simulink subsystem "Publish_Control_System_Out"  (R2023a)
settings: Solver=VariableStepAuto  StartTime=0.0  StopTime=10.0  RelTol=1e-3
undefined symbols (not defined in the file or in its folder): angular, data, data_SL_Info, linear
libraries: ros2lib x14
settings Model: Creator=hollis  LastModifiedBy=john

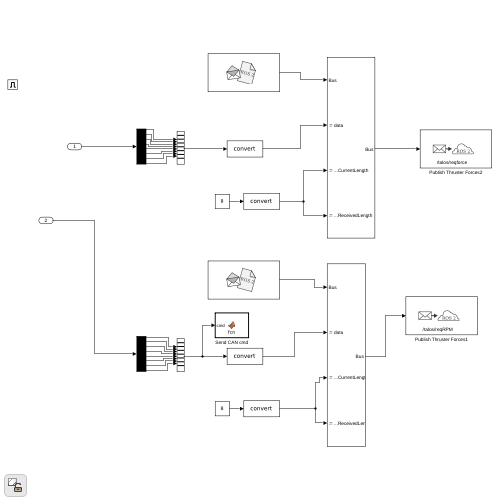
[thumbnail: Simulink's stored preview of the top-level diagram]
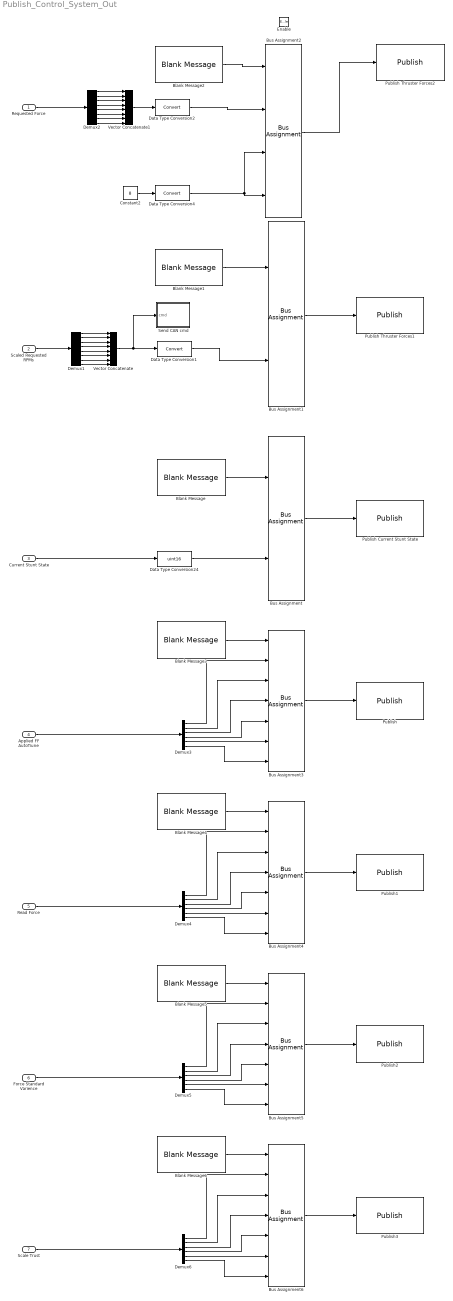
== system Publish_Control_System_Out ==
  Requested Force : Inport
  Scaled Requested RPMs : Inport  Port=2
  Current Stunt State : Inport  Port=3
  Applied FF AutoTiune : Inport  Port=4
  Read Force : Inport  Port=5
  Force Standard Varience : Inport  Port=6
  Scale Trust : Inport  Port=7
  Enable : EnablePort
  Blank Message : ros2lib/Blank Message  messageClass=Message  entityType=std_msgs/UInt16  messageType=std_msgs/UInt16  SampleTime=inf
  Blank Message1 : ros2lib/Blank Message  messageClass=Message  entityType=riptide_msgs2/DshotCommand  messageType=riptide_msgs2/DshotCommand  SampleTime=inf
      settings: LibrarySourceBlock=roslib/ROS 2/Blank Message
  Blank Message2 : ros2lib/Blank Message  messageClass=Message  entityType=std_msgs/Float32MultiArray  messageType=std_msgs/Float32MultiArray  SampleTime=inf
      settings: LibrarySourceBlock=roslib/ROS 2/Blank Message
  Blank Message{3..6} (4 alike) : ros2lib/Blank Message  messageClass=Message  entityType=geometry_msgs/Twist  messageType=geometry_msgs/Twist  SampleTime=inf
  Bus Assignment : BusAssignment  AssignedSignals=data
  Bus Assignment1 : BusAssignment  AssignedSignals=values
  Bus Assignment2 : BusAssignment  AssignedSignals=data,data_SL_Info.CurrentLength,data_SL_Info.ReceivedLength
  Bus Assignment{3..6} (4 alike) : BusAssignment  AssignedSignals=linear.x,linear.y,linear.z,angular.x,angular.y,angular.z
  Constant2 : Constant  Value=8
  Data Type Conversion1 : DataTypeConversion  SaturateOnIntegerOverflow=off  RndMeth=Floor
  Data Type Conversion2 : DataTypeConversion  SaturateOnIntegerOverflow=off  RndMeth=Floor
  Data Type Conversion24 : DataTypeConversion  OutDataTypeStr=uint16  SaturateOnIntegerOverflow=off  RndMeth=Floor
  Data Type Conversion4 : DataTypeConversion  SaturateOnIntegerOverflow=off  RndMeth=Floor
  Demux1 : Demux  Outputs=8
  Demux2 : Demux  Outputs=8
  Demux{3..6} (4 alike) : Demux  Outputs=6
  Publish : ros2lib/Publish  topicSource=Specify your own  topic=/talos/ff_auto_tune  messageType=geometry_msgs/Twist  QOSHistory=Keep last  QOSDepth=1  QOSReliability=Reliable  QOSDurability=Volatile
  Publish Current Stunt State : ros2lib/Publish  topicSource=Specify your own  topic=/talos/controller/running_stunt_state  messageType=std_msgs/UInt16  QOSHistory=Keep last  QOSDepth=1  QOSReliability=Reliable  QOSDurability=Volatile
  Publish Thruster Forces1 : ros2lib/Publish  topicSource=Specify your own  topic=/talos/command/requested_rpm  messageType=riptide_msgs2/DshotCommand  QOSHistory=Keep last  QOSDepth=1  QOSReliability=Reliable  QOSDurability=Volatile
      settings: LibrarySourceBlock=roslib/ROS 2/Publish
  Publish Thruster Forces2 : ros2lib/Publish  topicSource=Specify your own  topic=/talos/thruster_forces  messageType=std_msgs/Float32MultiArray  QOSHistory=Keep last  QOSDepth=1  QOSReliability=Reliable  QOSDurability=Volatile
      settings: LibrarySourceBlock=roslib/ROS 2/Publish
  Publish1 : ros2lib/Publish  topicSource=Specify your own  topic=/talos/controller/scale/applied_force_reading  messageType=geometry_msgs/Twist  QOSHistory=Keep last  QOSDepth=1  QOSReliability=Reliable  QOSDurability=Volatile
  Publish2 : ros2lib/Publish  topicSource=Specify your own  topic=/talos/controller/scale/standard_variance  messageType=geometry_msgs/Twist  QOSHistory=Keep last  QOSDepth=1  QOSReliability=Reliable  QOSDurability=Volatile
  Publish3 : ros2lib/Publish  topicSource=Specify your own  topic=/talos/controller/scale/trust  messageType=geometry_msgs/Twist  QOSHistory=Keep last  QOSDepth=1  QOSReliability=Reliable  QOSDurability=Volatile
  Send CAN cmd : MATLAB Function  TreatAsAtomicUnit=on
  Vector Concatenate : Concatenate  NumInputs=8
  Vector Concatenate1 : Concatenate  NumInputs=8
  wires:
  Demux1/8 -> Vector Concatenate/8
  Data Type Conversion2/1 -> Bus Assignment2/2
  Demux1/1 -> Vector Concatenate/1
  Demux2/4 -> Vector Concatenate1/4
  Demux2/5 -> Vector Concatenate1/5
  Demux2/2 -> Vector Concatenate1/2
  Blank Message2/1 -> Bus Assignment2/1
  Demux2/7 -> Vector Concatenate1/7
  Demux1/2 -> Vector Concatenate/2
  Constant2/1 -> Data Type Conversion4/1
  Blank Message1/1 -> Bus Assignment1/1
  Demux2/3 -> Vector Concatenate1/3
  Demux1/6 -> Vector Concatenate/6
  Scaled Requested RPMs/1 -> Demux1/1
  Data Type Conversion4/1 -> Bus Assignment2/4, Bus Assignment2/3
  Vector Concatenate1/1 -> Data Type Conversion2/1
  Demux1/4 -> Vector Concatenate/4
  Vector Concatenate/1 -> Send CAN cmd/1(cmd), Data Type Conversion1/1
  Demux1/5 -> Vector Concatenate/5
  Demux1/3 -> Vector Concatenate/3
  Demux2/8 -> Vector Concatenate1/8
  Demux2/6 -> Vector Concatenate1/6
  Demux1/7 -> Vector Concatenate/7
  Bus Assignment1/1 -> Publish Thruster Forces1/1
  Requested Force/1 -> Demux2/1
  Data Type Conversion1/1 -> Bus Assignment1/2
  Demux2/1 -> Vector Concatenate1/1
  Blank Message/1 -> Bus Assignment/1
  Bus Assignment/1 -> Publish Current Stunt State/1
  Current Stunt State/1 -> Data Type Conversion24/1
  Data Type Conversion24/1 -> Bus Assignment/2
  Applied FF AutoTiune/1 -> Demux3/1
  Demux3/6 -> Bus Assignment3/7
  Blank Message3/1 -> Bus Assignment3/1
  Bus Assignment3/1 -> Publish/1
  Demux3/1 -> Bus Assignment3/2
  Demux3/2 -> Bus Assignment3/3
  Demux3/4 -> Bus Assignment3/5
  Demux3/5 -> Bus Assignment3/6
  Demux3/3 -> Bus Assignment3/4
  Read Force/1 -> Demux4/1
  Blank Message4/1 -> Bus Assignment4/1
  Demux4/6 -> Bus Assignment4/7
  Demux4/2 -> Bus Assignment4/3
  Bus Assignment4/1 -> Publish1/1
  Demux4/1 -> Bus Assignment4/2
  Demux4/4 -> Bus Assignment4/5
  Demux4/5 -> Bus Assignment4/6
  Demux4/3 -> Bus Assignment4/4
  Force Standard Varience/1 -> Demux5/1
  Blank Message5/1 -> Bus Assignment5/1
  Demux5/6 -> Bus Assignment5/7
  Demux5/2 -> Bus Assignment5/3
  Bus Assignment5/1 -> Publish2/1
  Demux5/1 -> Bus Assignment5/2
  Demux5/4 -> Bus Assignment5/5
  Demux5/5 -> Bus Assignment5/6
  Demux5/3 -> Bus Assignment5/4
  Demux6/3 -> Bus Assignment6/4
  Demux6/4 -> Bus Assignment6/5
  Demux6/2 -> Bus Assignment6/3
  Demux6/5 -> Bus Assignment6/6
  Demux6/6 -> Bus Assignment6/7
  Demux6/1 -> Bus Assignment6/2
  Bus Assignment6/1 -> Publish3/1
  Blank Message6/1 -> Bus Assignment6/1
  Scale Trust/1 -> Demux6/1
  Bus Assignment2/1 -> Publish Thruster Forces2/1

== matlab function Publish_Control_System_Out/Send CAN cmd ==
  data: cmd input
function fcn(cmd)
send_thruster_cmd(cmd);
